simulink model "Assignment_V_Simulink"  (R2024b)
settings: Solver=FixedStepAuto  StartTime=0.0  StopTime=200  FixedStep=1/30  RelTol=1e-3
settings Model: Creator=vigno  LastModifiedBy=vigno

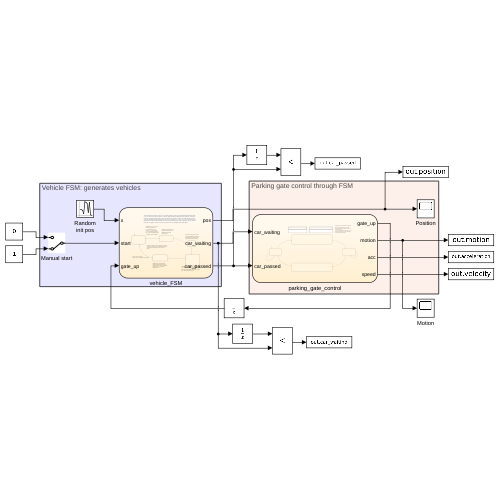
[thumbnail: Simulink's stored preview of the top-level diagram]
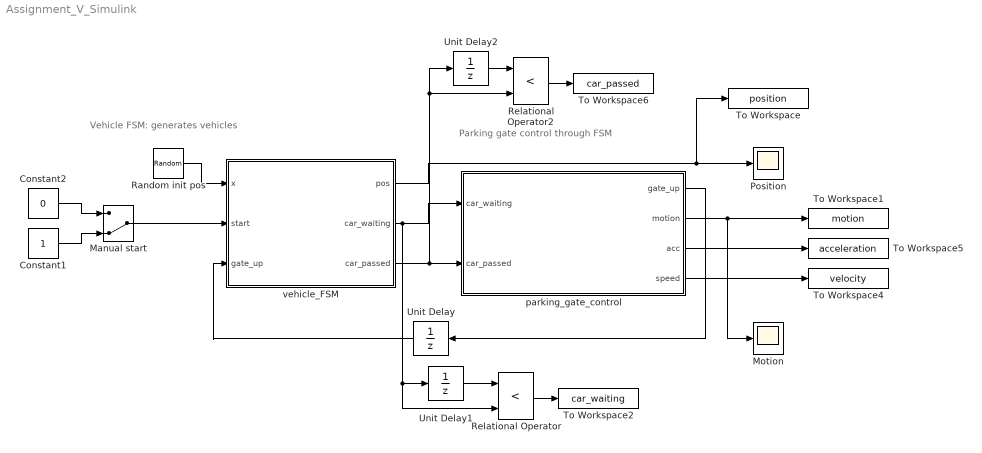
== system Assignment_V_Simulink ==
  note: Parking gate control through FSM
  note: Vehicle FSM: generates vehicles
  Constant1 : Constant
  Constant2 : Constant  Value=0
  Manual start : ManualSwitch  CurrentSetting=0
  Motion : Scope
  Position : Scope
  Random init pos : RandomNumber  Mean=-15  Variance=5  SampleTime=1/30
  Relational Operator : RelationalOperator  Operator=<  OutDataTypeStr=boolean  RndMeth=Simplest  InputSameDT=off
  Relational Operator2 : RelationalOperator  Operator=<  OutDataTypeStr=boolean  RndMeth=Simplest  InputSameDT=off
  To Workspace : ToWorkspace  VariableName=position  SaveFormat=Timeseries  SampleTime=-1
  To Workspace1 : ToWorkspace  VariableName=motion  SaveFormat=Timeseries  SampleTime=-1
  To Workspace2 : ToWorkspace  VariableName=car_waiting  SaveFormat=Timeseries  SampleTime=-1
  To Workspace4 : ToWorkspace  VariableName=velocity  SaveFormat=Timeseries  SampleTime=-1
  To Workspace5 : ToWorkspace  VariableName=acceleration  SaveFormat=Timeseries  SampleTime=-1
  To Workspace6 : ToWorkspace  VariableName=car_passed  SaveFormat=Timeseries  SampleTime=-1
  Unit Delay : UnitDelay  SampleTime=-1  HasFrameUpgradeWarning=on
  Unit Delay1 : UnitDelay  SampleTime=-1  HasFrameUpgradeWarning=on
  Unit Delay2 : UnitDelay  SampleTime=-1  HasFrameUpgradeWarning=on
  parking_gate_control : Stateflow chart  TreatAsAtomicUnit=on
  vehicle_FSM : Stateflow chart  TreatAsAtomicUnit=on
  wires:
  Constant1/1 -> Manual start/2
  Random init pos/1 -> vehicle_FSM/1(x)
  Constant2/1 -> Manual start/1
  Manual start/1 -> vehicle_FSM/2(start)
  vehicle_FSM/1(pos) -> To Workspace/1, Position/1
  vehicle_FSM/2(car_waiting) -> Relational Operator/2, Unit Delay1/1, parking_gate_control/1(car_waiting)
  vehicle_FSM/3(car_passed) -> Unit Delay2/1, Relational Operator2/2, parking_gate_control/2(car_passed)
  parking_gate_control/1(gate_up) -> Unit Delay/1
  Unit Delay/1 -> vehicle_FSM/3(gate_up)
  Unit Delay1/1 -> Relational Operator/1
  Relational Operator/1 -> To Workspace2/1
  Unit Delay2/1 -> Relational Operator2/1
  Relational Operator2/1 -> To Workspace6/1
  parking_gate_control/2(motion) -> Motion/1, To Workspace1/1
  parking_gate_control/3(acc) -> To Workspace5/1
  parking_gate_control/4(speed) -> To Workspace4/1

== stateflow chart Assignment_V_Simulink/parking_gate_control ==
  note: As the gate is up only when completely lifted, it becomes down even at the beginning (red traffic light in real life, as in the simulation).
      | To do so, we simply choose gate_up==0 from the beginning, but with a variable red_light to keep closing it.
  state raising
    [motion, speed, acc, gate_up] = custom_raise(elapsed(sec));
    t = elapsed(sec);
    % Returns gate_up and the actual motion, in particular from the elapsed_time, using a simple
    % motion law (from the initial position, velocity rising to the maximum, constant, decelerating to 90).
  state down
    gate_up=0;
    % Angular position of gate.
  state up
    % car_passed provided as
    % an input: wait until it's true.
  state lowering
    [motion, speed, acc, gate_up, red_light] = custom_lower(elapsed(sec));
    t = elapsed(sec);
    % Returns gate_up and the actual motion, in particular from the elapsed_time, using a simple
    % motion law (from the initial position, velocity rising to the maximum, constant, decelerating to 0).
    % From the beginning, activates a red light (traffic light) avoiding the cars to go on.
  down -> raising [order 2] : [car_waiting==1]
  raising -> up : [gate_up==1]
  (default) -> down
  up -> up [order 1] : [car_passed==0]
  down -> down [order 1] : [car_waiting==0]
  up -> lowering [order 2] : [car_passed==1]
  lowering -> down : [gate_up==0 && red_light ==0]
  data: time function_input; pos function_output; speed function_output; acc function_output; flag function_output; time function_input; pos function_output; speed function_output; acc function_output; flag function_output; red_flag function_output; car_waiting input; car_passed input; gate_up output; motion output; max_speed constant double =4; max_acc_dec constant double =1; t local; red_light local; acc output; speed output
  function [pos, speed, acc, flag] = custom_raise(time):
    | function [pos, speed, acc, flag] = custom_raise(time)
    | %#codegen
    | 
    |     if time < 4
    |         % First part, when we accelerate.
    |         pos = 1/2 * max_acc_dec * time^2;
    |         speed = max_acc_dec * time;
    |         acc = max_acc_dec;
    |     elseif time < 22.5
    |         % Second part, constant velocity (starting from 8°, 4s).
    |         pos = 8 + max_speed * (time - 4);
    |         speed = max_speed;
    |         acc = 0;
    |     else
    |         % Third part, starting from 82° and decelerating.
    |         pos = 82 + max_speed * (time - 22.5) - 1/2 * max_acc_dec * (time - 22.5)^2;
    |         speed = max_speed - max_acc_dec * (time - 22.5);
    |         acc = -max_acc_dec;
    |     end
    | 
    |     if time > 26.5
    |         flag = 1;
    |         pos = 90;
    |         speed = 0;
    |         acc = 0;
    |     else
    |         flag = 0;
    |     end
    | end
  function [pos, speed, acc, flag, red_flag] = custom_lower(time):
    | function [pos, speed, acc, flag, red_flag] = custom_lower(time)
    | %#codegen
    | 
    |     pos = 90;
    |     flag = 0;
    |     red_flag = 1;
    | 
    |     if time < 4
    |         % First part, when we accelerate.
    |         pos = 90 - 1/2 * max_acc_dec * time^2;
    |         speed = -max_acc_dec * time;
    |         acc = -max_acc_dec;
    |     elseif time < 22.5
    |         % Second part, constant velocity (starting from 82°, 4s).
    |         pos = 90 - 8 - max_speed * (time - 4);
    |         speed = -max_speed;
    |         acc = 0;
    |     else
    |         % Third part, starting from 82° and decelerating.
    |         pos = 8 - max_speed * (time - 22.5) + 1/2 * max_acc_dec * (time - 22.5)^2;
    |         speed = -max_speed + max_acc_dec * (time - 22.5);
    |         acc = max_acc_dec;
    |     end
    | 
    |     if time > 26.5
    |         red_flag = 0;
    |         pos = 0;
    |         speed = 0;
    |         acc = 0;
    |     end
    | end

== stateflow chart Assignment_V_Simulink/vehicle_FSM ==
  note: This continuously creates a new car in a random position, from a gaussian distribution having mean (-15). v is the car's velocity, which is constant, while position is adjourned every time the car moves. Gate has a physical length (gate_end). The outputs area position, which has to be plotted, and two flags (car_waiting and car_passed). As soon as car_waiting==1, i.e. pos >= 0, we can bring the gate up (before it is not suitable, because we can't know!). After the gate is up (input gate_up==1) we can move the car again; as soon as the car is passed, we can bring the gate down again!
  note: Initialization: init is x, pos too, while car_waiting and car_passed are put to 0.
      | If start == 1, we just keep pos=x, Gaussian rnd signal.
      | Pos is wrt the waiting position (if positive, we are waiting).
  note: Approaching: position (pos) starts from init (Gaussian signal) and increases linearly with v.
  note: We need to have gate_up true from the beginning to let the car passed, and it is given only as input (from a function output)
  state idle
    init=x;
    pos=init;
    car_waiting=0;
    car_passed=0;
  state approaching
    pos=init+v*elapsed(sec);
  state stop
    tmp=pos;
    car_waiting=1;
    car_passed=0;
  note: After 10 seconds, a new car arrives (new input x, random, which is also the position). We go on continuously creating new cars to have in queue.
  state pass
    pos=tmp+v*elapsed(sec);
    car_waiting=0;
    ex:
    pos=tmp+v*elapsed(sec);
    tmp=pos;
  state passed
    pos=tmp+v*elapsed(sec);
    car_passed=1;
  note: Input: x, start, gate_up
      | Output: pos, car_waiting, car_passed
  note: Variable gate_end shows the physical end's measure: when position is over, we get to passed and also flag car_passed is adjourned to 1.
  note: Since the gate is already up, we can pass with the car. Position is computed from the actual one, linearly with v then. At the exit, tmp is adjourned to pos.
  (default) -> idle
  approaching -> stop : [pos>=0]
  idle -> approaching : [start==1]
  passed -> idle : [after(10,sec)]
  stop -> pass : [gate_up==1]
  pass -> passed : [pos>= gate_end]
  data: gate_end local =3; v local double =1; pos output; car_waiting output; car_passed output; init local; x input; start input; gate_up input; tmp local
